simulink model "mainModel"  (R2024b)
settings: Solver=ode4  StartTime=0.0  StopTime=35000  FixedStep=0.1  RelTol=1e-3
values from neighbouring files (symbols this model uses):
  actuators = actuatorsConfig()    [main.m]
  constant = constantsConfig()    [main.m]
  control = controlConfig(data)    [main.m]
  MEKF = estimationConfig(sensors,simOpt)    [main.m]
  pert = pertConfig()    [main.m]
  sensors = sensorsConfig()    [main.m]
undefined symbols (not defined in the file or in its folder): Ab0, data, DiscIntNeverNeededParam, init
libraries: matrix_library x38, simulink x10, aerolibutil x7, simulink_extras x6, sharedtransform x1, dspinverses x1, dspfdesign x1, dspstat3 x1
(part 2 of 3)

== system mainModel/TRIAD/errorsTRIAD ==
  A_BN : Inport
  A_BN_est : Inport  Port=2
  w : Inport  Port=3
  w_estTRIAD : Inport  Port=4
  Minus1 : Sum  Inputs=+-
  Reshape : Reshape
  Scope : Scope
  Scope1 : Scope
  Scope2 : Scope
  Scope3 : Scope  NumInputPorts=2
  TRUE^t * SYM : Product  Multiplication=Matrix(*)
  To Workspace : ToWorkspace  VariableName=errTRIAD  SampleTime=-1
  Transpose : Math  Operator=transpose
  Zero-Order Hold : ZeroOrderHold  SampleTime=0.1
  Zero-Order Hold1 : ZeroOrderHold  SampleTime=0.1
  angle error : Subsystem
  wires:
  A_BN/1 -> Zero-Order Hold/1
  w/1 -> Zero-Order Hold1/1
  w_estTRIAD/1 -> Scope3/2, Minus1/2
  Minus1/1 -> Scope1/1
  TRUE^t * SYM/1 -> angle error/1(Aerr)
  angle error/1(theta_err) -> Reshape/1
  Transpose/1 -> TRUE^t * SYM/1
  A_BN_est/1 -> TRUE^t * SYM/2, Scope2/1
  Zero-Order Hold/1 -> Scope/1, Transpose/1
  Zero-Order Hold1/1 -> Scope3/1, Minus1/1
  Reshape/1 -> To Workspace/1

== system mainModel/angular rates estimation QUEST /angVelEstimation ==
  q_est : Inport
  Discrete-Time Integrator : DiscreteIntegrator  SampleTime=-1  ICPrevOutput=DiscIntNeverNeededParam  ICPrevScaledInput=DiscIntNeverNeededParam
  Gain : Gain  Gain=2
  Qmatrix : Subsystem  ReferencedSubsystem=Qmatrix
  Scope : Scope
  "[Q*] * q_dot" : Product  Multiplication=Matrix(*)
  pseudoInverseMatrix : Subsystem  ReferencedSubsystem=pseudoInverseMatrix
  w_est : Outport
  wires:
  q_est/1 -> Discrete-Time Integrator/1, Qmatrix/1
  Gain/1 -> Scope/1, w_est/1
  Discrete-Time Integrator/1 -> "[Q*] * q_dot"/2  "q_dot"
  "[Q*] * q_dot"/1 -> Gain/1
  Qmatrix/1 -> pseudoInverseMatrix/1
  pseudoInverseMatrix/1 -> "[Q*] * q_dot"/1

== system mainModel/angular rates estimation QUEST /svd ==
  K : Inport
  Dot Product : DotProduct  OutDataTypeStr=Inherit: Inherit via internal rule
  Gain : Gain  Gain=-1
  K * q : Product  Multiplication=Matrix(*)
  Memory : Memory  InitialCondition=init.q0
  Scope{,1..3} (4 alike) : Scope
  Subsystem Reference : Subsystem  ReferencedSubsystem=vecNorm
  Switch : Switch  Criteria=u2 > Threshold  SaturateOnIntegerOverflow=off  InputSameDT=off
  Terminator : Terminator
  To Workspace : ToWorkspace  VariableName=q_est_SVD  SampleTime=-1
  q_est : Outport
  wires:
  K/1 -> Scope1/1, K * q/1  "Kmatrix (4x4)"
  Subsystem Reference/2 -> Switch/1, Gain/1, Memory/1, Dot Product/1, Scope/1, Scope3/1, To Workspace/1, q_est/1  "q_optimal"
  Subsystem Reference/1 -> Terminator/1
  Memory/1 -> K * q/2, Dot Product/2  "qVec (4x1)"
  K * q/1 -> Subsystem Reference/1
  Dot Product/1 -> Switch/2
  Gain/1 -> Switch/3
  Switch/1 -> Scope2/1

== system mainModel/atmDrag/DRAG torque  ==
  rho : Inport
  velRel_B : Inport  Port=2
  w_B : Inport  Port=3
  Constant : Constant  Value=pert.drag.Nbvect
  Constant1 : Constant  Value=pert.drag.rF
  Constant2 : Constant  Value=pert.drag.A
  Relative velocity body : Subsystem
  To Workspace1 : ToWorkspace  VariableName=dragPertMatrix  SampleTime=-1
  dragForce : Subsystem
  dragTorque : Subsystem
  vecCrossOld : Subsystem  Commented=on
  DRAG : Outport
  wires:
  velRel_B/1 -> Relative velocity body/1(velRel_B)
  w_B/1 -> Relative velocity body/2(om_B)
  Constant1/1 -> Relative velocity body/3(rF), dragTorque/2(rFvect)
  Relative velocity body/1(vRelBody) -> dragForce/2(vRelBody)
  rho/1 -> dragForce/1(rho)
  Constant/1 -> dragForce/3(Nb)
  Constant2/1 -> dragForce/4(A)
  dragForce/1(F) -> dragTorque/1(Fvect)
  dragTorque/1(DRAG) -> DRAG/1
  dragTorque/2(dragMATRIX) -> To Workspace1/1

== system mainModel/atmDrag/density ==
  r_N : Inport
  Constant : Constant  Value=constant.Re
  Constant1 : Constant  Value=pert.drag.h0_vect
  Constant2 : Constant  Value=pert.drag.H_vect
  Constant4 : Constant  Value=pert.drag.rho0_vect
  Constant5 : Constant  Value=pert.drag.h0_vect
  Divide : Product  Inputs=*/
  Exp : Math
  Gain : Gain  Gain=-1
  Interpolation Using Prelookup : Interpolation_n-D  NumberOfTableDimensions=1  TableSource=Input port  InternalRulePriority=Speed
      settings: InputPortMap=u0,u1,p2
  Interpolation Using Prelookup1 : Interpolation_n-D  NumberOfTableDimensions=1  TableSource=Input port  InternalRulePriority=Speed
      settings: InputPortMap=u0,u1,p2
  Interpolation Using Prelookup2 : Interpolation_n-D  NumberOfTableDimensions=1  TableSource=Input port  InternalRulePriority=Speed
      settings: InputPortMap=u0,u1,p2
  Minus : Sum  Inputs=+-
  Minus1 : Sum  Inputs=+-
  Prelookup : PreLookup  BreakpointsDataSource=Input port  BreakpointsData=[10:10:110]  ExtrapMethod=Linear
      settings: InputPortMap=u0,p1
  Product : Product
  Subsystem Reference : Subsystem  ReferencedSubsystem=vecNorm
  Terminator : Terminator
  rho : Outport
  wires:
  r_N/1 -> Subsystem Reference/1
  Subsystem Reference/2 -> Terminator/1
  Subsystem Reference/1 -> Minus/1
  Constant/1 -> Minus/2
  Minus/1 -> Minus1/1, Prelookup/1  "h"
  Constant1/1 -> Prelookup/2
  Prelookup/1 -> Interpolation Using Prelookup/1, Interpolation Using Prelookup2/1, Interpolation Using Prelookup1/1
  Prelookup/2 -> Interpolation Using Prelookup/2, Interpolation Using Prelookup1/2, Interpolation Using Prelookup2/2
  Constant5/1 -> Interpolation Using Prelookup/3
  Constant2/1 -> Interpolation Using Prelookup1/3
  Constant4/1 -> Interpolation Using Prelookup2/3
  Interpolation Using Prelookup/1 -> Minus1/2
  Interpolation Using Prelookup1/1 -> Divide/2
  Minus1/1 -> Divide/1
  Divide/1 -> Gain/1
  Exp/1 -> Product/1
  Interpolation Using Prelookup2/1 -> Product/2
  Product/1 -> rho/1
  Gain/1 -> Exp/1

== system mainModel/atmDrag/relVel ==
  A_BN : Inport
  r_N : Inport  Port=2
  vel_N : Inport  Port=3
  A_BN * velRel_N : Product  Multiplication=Matrix(*)
  Add : Sum  Inputs=-+
  Constant : Constant  Value=[0;0;constant.we]  VectorParams1D=off
  Cross Product : matrix_library/Cross Product
  velRel_B : Outport
  wires:
  Constant/1 -> Cross Product/1
  r_N/1 -> Cross Product/2
  Cross Product/1 -> Add/1
  vel_N/1 -> Add/2
  Add/1 -> A_BN * velRel_N/2  "velRel_N"
  A_BN/1 -> A_BN * velRel_N/1
  A_BN * velRel_N/1 -> velRel_B/1

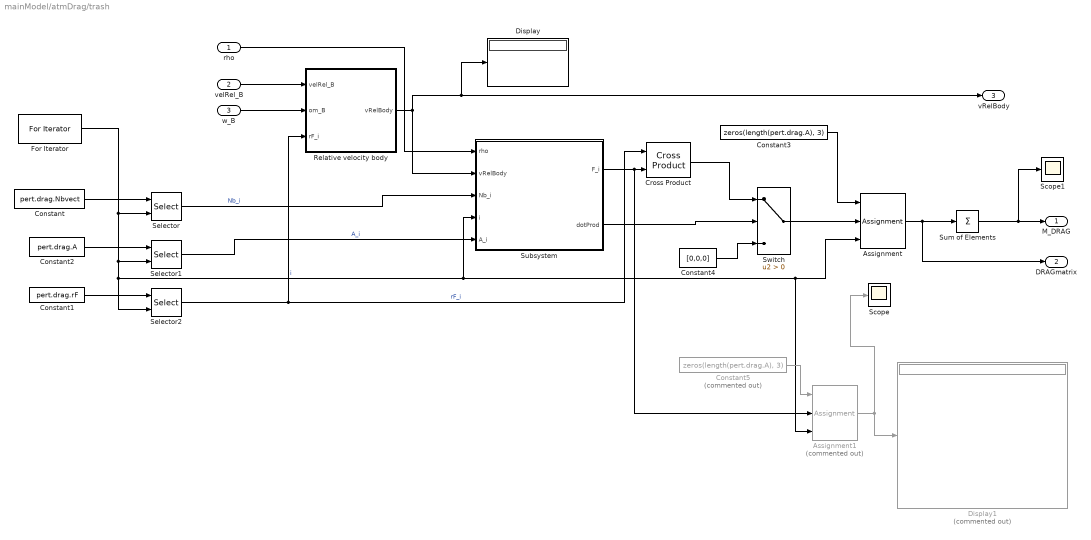
== system mainModel/atmDrag/trash ==
  rho : Inport
  velRel_B : Inport  Port=2
  w_B : Inport  Port=3
  Assignment : Assignment  NumberOfDimensions=2  DiagnosticForDimensions=Warning  IndexOptions=Index vector (port),Assign all  Indices=1,1  OutputSizes=1,1
  Assignment1 : Assignment  Commented=on  NumberOfDimensions=2  DiagnosticForDimensions=Warning  IndexOptions=Index vector (port),Assign all  Indices=1,1  OutputSizes=1,1
  Constant : Constant  Value=pert.drag.Nbvect
  Constant1 : Constant  Value=pert.drag.rF
  Constant2 : Constant  Value=pert.drag.A
  Constant3 : Constant  Value=zeros(length(pert.drag.A), 3)  VectorParams1D=off
  Constant4 : Constant  Value=[0,0,0]  VectorParams1D=off
  Constant5 : Constant  Commented=on  Value=zeros(length(pert.drag.A), 3)  VectorParams1D=off
  Cross Product : matrix_library/Cross Product
  Display : Display
  Display1 : Display  Commented=on
  For Iterator : ForIterator  IterationLimit=length(pert.drag.A)
  Relative velocity body : Subsystem
  Scope : Scope
  Scope1 : Scope
  Selector : Selector  NumberOfDimensions=2  InputPortWidth=3  IndexOptions=Index vector (port),Select all  Indices=[1 3],1  OutputSizes=1,1
  Selector1 : Selector  InputPortWidth=10  IndexOptions=Index vector (port)  Indices=[1 3]  OutputSizes=1
  Selector2 : Selector  NumberOfDimensions=2  InputPortWidth=3  IndexOptions=Index vector (port),Select all  Indices=[1 3],1  OutputSizes=1,1
  Subsystem : Subsystem
  Sum of Elements : Sum  Inputs=+  CollapseMode=Specified dimension
  Switch : Switch  Criteria=u2 > Threshold  SaturateOnIntegerOverflow=off  InputSameDT=off
  M_DRAG : Outport
  DRAGmatrix : Outport  Port=2
  vRelBody : Outport  Port=3
  wires:
  Constant/1 -> Selector/1
  Constant2/1 -> Selector1/1
  Constant1/1 -> Selector2/1
  Selector2/1 -> Relative velocity body/3(rF_i), Cross Product/1  "rF_i"
  For Iterator/1 -> Selector2/2, Subsystem/4(i), Assignment1/3, Assignment/3, Selector1/2, Selector/2  "i"
  Cross Product/1 -> Switch/1
  rho/1 -> Subsystem/1(rho)
  velRel_B/1 -> Relative velocity body/1(velRel_B)
  Selector/1 -> Subsystem/3(Nb_i)  "Nb_i"
  Selector1/1 -> Subsystem/5(A_i)  "A_i"
  Subsystem/1(F_i) -> Assignment1/2, Cross Product/2
  Assignment/1 -> Sum of Elements/1, DRAGmatrix/1
  Relative velocity body/1(vRelBody) -> Display/1, vRelBody/1, Subsystem/2(vRelBody)
  Sum of Elements/1 -> Scope1/1, M_DRAG/1
  Constant3/1 -> Assignment/1
  Subsystem/2(dotProd) -> Switch/2
  Constant4/1 -> Switch/3
  Switch/1 -> Assignment/2
  w_B/1 -> Relative velocity body/2(om_B)
  Constant5/1 -> Assignment1/1
  Assignment1/1 -> Scope/1, Display1/1

== system mainModel/attitudeDetermination_QUATERNION/QUEST ==
  S : Inport
  z : Inport  Port=2
  sigma : Inport  Port=3
  -z * [S-(sigma+1)*I]^-1 : Product  Multiplication=Matrix(*)
  Add : Sum
  Add1 : Sum
  Constant : Constant  Value=init.lambda0
  Constant1 : Constant  Value=eye(3)
  Gain : Gain  Gain=-1
  Gain1 : Gain  Gain=-1
  Product : Product
  Scope3 : Scope
  Subsystem Reference : Subsystem  ReferencedSubsystem=invertMatrix
  Subsystem Reference1 : Subsystem  ReferencedSubsystem=quat2DCM
  To Workspace : ToWorkspace  VariableName=q_est_QUESTgibbs  SampleTime=-1
  fix quat : Subsystem  ReferencedSubsystem=quatFix
  gibbs2quat : Subsystem  ReferencedSubsystem=gibbs2quat
  q_est : Outport
  wires:
  sigma/1 -> Add/1
  Add/1 -> Product/1  "sigma + 1"
  Constant1/1 -> Product/2
  Product/1 -> Gain/1
  Gain/1 -> Add1/2  "-(sigma+1)*I"
  S/1 -> Add1/1  "S"
  Subsystem Reference/1 -> -z * [S-(sigma+1)*I]^-1/1
  z/1 -> Gain1/1
  -z * [S-(sigma+1)*I]^-1/1 -> gibbs2quat/1  "gibbs_est"
  Gain1/1 -> -z * [S-(sigma+1)*I]^-1/2
  gibbs2quat/1 -> fix quat/1  "q_prev"
  fix quat/1 -> Subsystem Reference1/1, To Workspace/1, q_est/1
  Constant/1 -> Add/2
  Add1/1 -> Subsystem Reference/1
  Subsystem Reference1/1 -> Scope3/1

== system mainModel/attitudeDetermination_QUATERNION/QUEST V2 ==
  z : Inport
  sigma : Inport  Port=2
  S : Inport  Port=3
  Add : Sum
  Constant : Constant  Value=eye(3)
  Constant1 : Constant  Value=init.lambda0
  Minus : Sum  Inputs=+-
  Product : Product
  Product1 : Product  Multiplication=Matrix(*)
  Scope1 : Scope
  Subsystem Reference : Subsystem  ReferencedSubsystem=matrixDeterminant
  Subsystem Reference2 : Subsystem  ReferencedSubsystem=vecNorm
  Subsystem Reference3 : Subsystem  ReferencedSubsystem=quat2DCM
  Terminator : Terminator
  To Workspace1 : ToWorkspace  VariableName=q_est_QUESTadj  SampleTime=-1
  Vector Concatenate : Concatenate
  adjointMatrix : Subsystem
  q_est : Outport
  wires:
  sigma/1 -> Add/1
  Add/1 -> Product/2  "rho"
  Constant/1 -> Product/1
  Constant1/1 -> Add/2
  Product/1 -> Minus/1  "rho*I"
  S/1 -> Minus/2
  Minus/1 -> Subsystem Reference/1, adjointMatrix/1(A)
  z/1 -> Product1/2
  Product1/1 -> Vector Concatenate/1
  Subsystem Reference/1 -> Vector Concatenate/2
  Vector Concatenate/1 -> Subsystem Reference2/1
  Subsystem Reference2/2 -> To Workspace1/1, q_est/1, Subsystem Reference3/1
  Subsystem Reference3/1 -> Scope1/1
  adjointMatrix/1(Out1) -> Product1/1
  Subsystem Reference2/1 -> Terminator/1

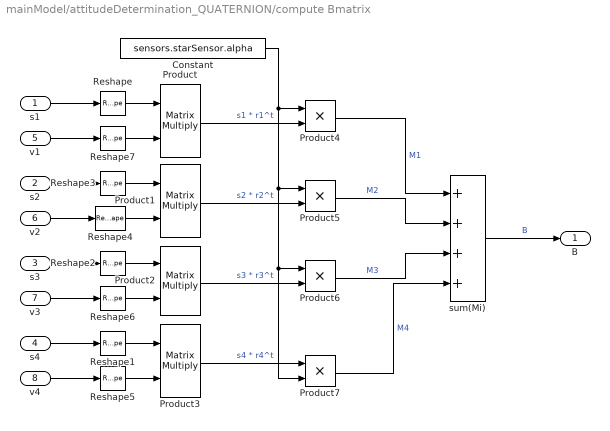
== system mainModel/attitudeDetermination_QUATERNION/compute Bmatrix ==
  s1 : Inport
  s2 : Inport  Port=2
  s3 : Inport  Port=3
  s4 : Inport  Port=4
  v1 : Inport  Port=5
  v2 : Inport  Port=6
  v3 : Inport  Port=7
  v4 : Inport  Port=8
  Constant : Constant  Value=sensors.starSensor.alpha
  Product{,1..3} (4 alike) : Product  Multiplication=Matrix(*)
  Product{4..7} (4 alike) : Product
  Reshape{,1..3} (4 alike) : Reshape  OutputDimensionality=Column vector (2-D)
  Reshape{4..7} (4 alike) : Reshape  OutputDimensionality=Row vector (2-D)
  sum(Mi) : Sum  Inputs=++++
  B : Outport
  wires:
  sum(Mi)/1 -> B/1  "B"
  Product/1 -> Product4/2  "s1 * r1^t"
  Constant/1 -> Product4/1, Product5/1, Product7/2, Product6/1
  Product1/1 -> Product5/2  "s2 * r2^t"
  Product2/1 -> Product6/2  "s3 * r3^t"
  Product3/1 -> Product7/1  "s4 * r4^t"
  Product4/1 -> sum(Mi)/1  "M1"
  Product6/1 -> sum(Mi)/3  "M3"
  Product5/1 -> sum(Mi)/2  "M2"
  Reshape4/1 -> Product1/2
  Reshape1/1 -> Product3/1
  Reshape/1 -> Product/1
  Reshape2/1 -> Product2/1
  Reshape6/1 -> Product2/2
  Reshape7/1 -> Product/2
  Reshape5/1 -> Product3/2
  v4/1 -> Reshape5/1
  v2/1 -> Reshape4/1
  v1/1 -> Reshape7/1
  s1/1 -> Reshape/1
  Reshape3/1 -> Product1/1
  v3/1 -> Reshape6/1
  s4/1 -> Reshape1/1
  s3/1 -> Reshape2/1
  Product7/1 -> sum(Mi)/4  "M4"
  s2/1 -> Reshape3/1

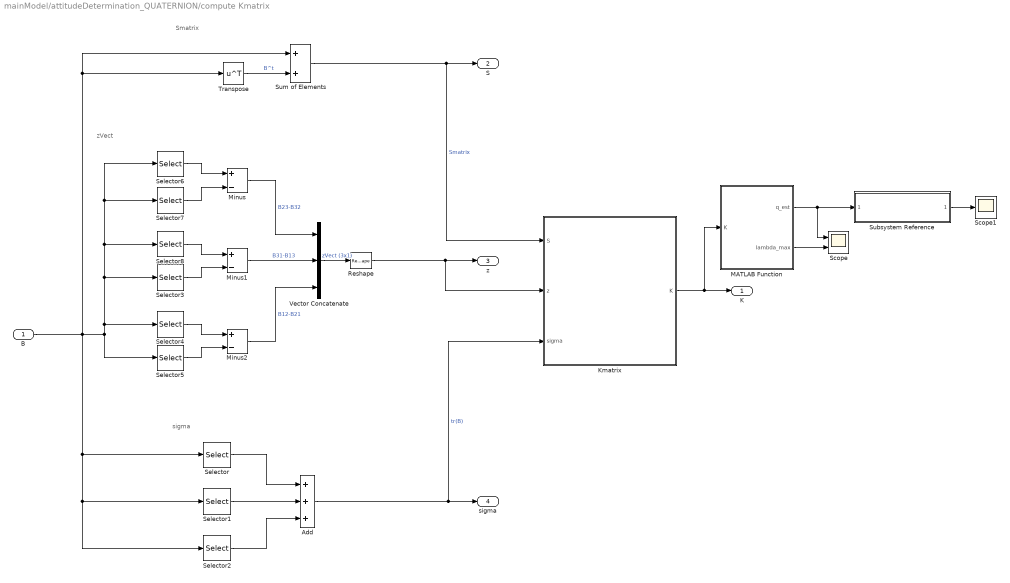
== system mainModel/attitudeDetermination_QUATERNION/compute Kmatrix ==
  note: Smatrix
  note: zVect
  note: sigma
  B : Inport
  Add : Sum  Inputs=+++
  Kmatrix : Subsystem
  MATLAB Function : MATLAB Function  TreatAsAtomicUnit=on
  Minus : Sum  Inputs=+-
  Minus1 : Sum  Inputs=+-
  Minus2 : Sum  Inputs=+-
  Reshape : Reshape  OutputDimensionality=Column vector (2-D)
  Scope : Scope  NumInputPorts=2
  Scope1 : Scope
  Selector : Selector  NumberOfDimensions=2  InputPortWidth=3  IndexOptions=Index vector (dialog),Index vector (dialog)  Indices=1,1  OutputSizes=1,1
  Selector1 : Selector  NumberOfDimensions=2  InputPortWidth=3  IndexOptions=Index vector (dialog),Index vector (dialog)  Indices=2,2  OutputSizes=1,1
  Selector2 : Selector  NumberOfDimensions=2  InputPortWidth=3  IndexOptions=Index vector (dialog),Index vector (dialog)  Indices=3,3  OutputSizes=1,1
  Selector3 : Selector  NumberOfDimensions=2  InputPortWidth=3  IndexOptions=Index vector (dialog),Index vector (dialog)  Indices=1,3  OutputSizes=1,1
  Selector4 : Selector  NumberOfDimensions=2  InputPortWidth=3  IndexOptions=Index vector (dialog),Index vector (dialog)  Indices=1,2  OutputSizes=1,1
  Selector5 : Selector  NumberOfDimensions=2  InputPortWidth=3  IndexOptions=Index vector (dialog),Index vector (dialog)  Indices=2,1  OutputSizes=1,1
  Selector6 : Selector  NumberOfDimensions=2  InputPortWidth=3  IndexOptions=Index vector (dialog),Index vector (dialog)  Indices=2,3  OutputSizes=1,1
  Selector7 : Selector  NumberOfDimensions=2  InputPortWidth=3  IndexOptions=Index vector (dialog),Index vector (dialog)  Indices=3,2  OutputSizes=1,1
  Selector8 : Selector  NumberOfDimensions=2  InputPortWidth=3  IndexOptions=Index vector (dialog),Index vector (dialog)  Indices=3,1  OutputSizes=1,1
  Subsystem Reference : Subsystem  ReferencedSubsystem=quat2DCM
  Sum of Elements : Sum
  Transpose : Math  Operator=transpose
  Vector Concatenate : Concatenate  NumInputs=3
  K : Outport
  S : Outport  Port=2
  z : Outport  Port=3
  sigma : Outport  Port=4
  wires:
  Reshape/1 -> Kmatrix/2(z), z/1
  Kmatrix/1(K) -> MATLAB Function/1(K), K/1
  Add/1 -> Kmatrix/3(sigma), sigma/1  "tr(B)"
  Selector2/1 -> Add/3
  Selector/1 -> Add/1
  Selector1/1 -> Add/2
  Vector Concatenate/1 -> Reshape/1  "zVect (3x1)"
  Minus2/1 -> Vector Concatenate/3  "B12-B21"
  Minus/1 -> Vector Concatenate/1  "B23-B32"
  Minus1/1 -> Vector Concatenate/2  "B31-B13"
  Selector4/1 -> Minus2/1
  Selector5/1 -> Minus2/2
  Selector8/1 -> Minus1/1
  Selector3/1 -> Minus1/2
  Selector7/1 -> Minus/2
  Selector6/1 -> Minus/1
  Transpose/1 -> Sum of Elements/2  "B^t"
  B/1 -> Selector2/1, Selector1/1, Selector/1, Selector3/1, Selector8/1, Selector7/1, Selector6/1, Selector4/1, Selector5/1, Transpose/1, Sum of Elements/1
  Sum of Elements/1 -> S/1, Kmatrix/1(S)  "Smatrix"
  MATLAB Function/1(q_est) -> Subsystem Reference/1, Scope/1
  MATLAB Function/2(lambda_max) -> Scope/2
  Subsystem Reference/1 -> Scope1/1

== system mainModel/attitudeDetermination_QUATERNION/matlaFunction for Davenport's q-method ==
  K : Inport
  MATLAB Function : MATLAB Function  TreatAsAtomicUnit=on
  Reshape : Reshape
  Reshape1 : Reshape
  To Workspace : ToWorkspace  VariableName=lambdaMax_DavqMethod  SampleTime=-1
  To Workspace3 : ToWorkspace  VariableName=q_est_DavqMethod  SampleTime=-1
  q_est : Outport
  lambda_max : Outport  Port=2
  wires:
  MATLAB Function/1(q_est) -> q_est/1, Reshape1/1
  K/1 -> MATLAB Function/1(K)
  MATLAB Function/2(lambda_max) -> lambda_max/1, Reshape/1
  Reshape/1 -> To Workspace/1
  Reshape1/1 -> To Workspace3/1

== system mainModel/attitudeDetermination_QUATERNION/quest - shuster ==
  note: compute MAX eigenvalue
  S : Inport
  z : Inport  Port=2
  Constant : Constant  Value=init.lambda0
  Reshape : Reshape
  Scope1 : Scope
  Scope2 : Scope
  Subsystem Reference : Subsystem  ReferencedSubsystem=quat2DCM
  To Workspace : ToWorkspace  VariableName=lambdaMax_QUESTshuster  SampleTime=-1
  To Workspace2 : ToWorkspace  VariableName=q_est_QUESTshuster  SampleTime=-1
  compute optimal quaternion : Subsystem
  mewton method step-two : Subsystem  Commented=on
  newton method step-one : Subsystem
  shuster parameters : Subsystem
  q_est : Outport
  lambda : Outport  Port=2
  wires:
  compute optimal quaternion/1(q_est) -> Scope1/1, To Workspace2/1, Subsystem Reference/1, q_est/1
  Reshape/1 -> compute optimal quaternion/1(lambda), lambda/1, To Workspace/1
  S/1 -> compute optimal quaternion/5(S), shuster parameters/1(S)  "S"
  z/1 -> compute optimal quaternion/6(z), shuster parameters/2(z)  "z"
  shuster parameters/6(k) -> compute optimal quaternion/3(k)
  shuster parameters/7(Delta) -> compute optimal quaternion/4(Delta)
  Subsystem Reference/1 -> Scope2/1
  newton method step-one/1(lambda1) -> Reshape/1
  Constant/1 -> newton method step-one/1(lambda)
  shuster parameters/4(d) -> newton method step-one/6(d)
  shuster parameters/3(c) -> newton method step-one/5(c)
  shuster parameters/2(b) -> newton method step-one/4(b)
  shuster parameters/1(a) -> newton method step-one/3(a)
  shuster parameters/5(sigma) -> newton method step-one/2(sigma), compute optimal quaternion/2(sigma)

== system mainModel/attitudeError/angle error ==
  Aerr : Inport
  Acos : Trigonometry  Operator=acos
  Add : Sum  Inputs=+++
  Constant : Constant
  Gain : Gain  Gain=1/2
  Minus1 : Sum  Inputs=+-
  Radians to Degrees : simulink_extras/Transformations/Radians to Degrees
  Selector : Selector  NumberOfDimensions=2  InputPortWidth=3  IndexOptions=Index vector (dialog),Index vector (dialog)  Indices=1,1  OutputSizes=1,1
  Selector1 : Selector  NumberOfDimensions=2  InputPortWidth=3  IndexOptions=Index vector (dialog),Index vector (dialog)  Indices=2,2  OutputSizes=1,1
  Selector2 : Selector  NumberOfDimensions=2  InputPortWidth=3  IndexOptions=Index vector (dialog),Index vector (dialog)  Indices=3,3  OutputSizes=1,1
  theta_err : Outport
  wires:
  Aerr/1 -> Selector2/1, Selector/1, Selector1/1
  Gain/1 -> Acos/1
  Selector1/1 -> Add/2
  Add/1 -> Minus1/1  "tr(Aerr)"
  Constant/1 -> Minus1/2
  Selector2/1 -> Add/3
  Minus1/1 -> Gain/1
  Selector/1 -> Add/1
  Acos/1 -> Radians to Degrees/1
  Radians to Degrees/1 -> theta_err/1

== system mainModel/attitudeError1/angle error ==
  Aerr : Inport
  Acos : Trigonometry  Operator=acos
  Add : Sum  Inputs=+++
  Constant : Constant
  Gain : Gain  Gain=1/2
  Minus1 : Sum  Inputs=+-
  Radians to Degrees : simulink_extras/Transformations/Radians to Degrees
  Reshape : Reshape
  Selector : Selector  NumberOfDimensions=2  InputPortWidth=3  IndexOptions=Index vector (dialog),Index vector (dialog)  Indices=1,1  OutputSizes=1,1
  Selector1 : Selector  NumberOfDimensions=2  InputPortWidth=3  IndexOptions=Index vector (dialog),Index vector (dialog)  Indices=2,2  OutputSizes=1,1
  Selector2 : Selector  NumberOfDimensions=2  InputPortWidth=3  IndexOptions=Index vector (dialog),Index vector (dialog)  Indices=3,3  OutputSizes=1,1
  theta_err : Outport
  wires:
  Aerr/1 -> Selector2/1, Selector/1, Selector1/1
  Gain/1 -> Acos/1
  Selector1/1 -> Add/2
  Add/1 -> Minus1/1  "tr(Aerr)"
  Constant/1 -> Minus1/2
  Selector2/1 -> Add/3
  Minus1/1 -> Gain/1
  Selector/1 -> Add/1
  Acos/1 -> Radians to Degrees/1
  Radians to Degrees/1 -> Reshape/1
  Reshape/1 -> theta_err/1

== system mainModel/basicMagModel/mHat ==
  we : Inport
  magAxAngle : Inport  Port=2
  Clock : Clock
  Cos : Trigonometry
  Cos1 : Trigonometry  Operator=cos
  Cos2 : Trigonometry
  Cos3 : Trigonometry  Operator=cos
  Product : Product
  Product1 : Product
  Product2 : Product
  Vector Concatenate : Concatenate  NumInputs=3
  mHat : Outport
  wires:
  Vector Concatenate/1 -> mHat/1
  Clock/1 -> Product/2
  Product/1 -> Cos2/1, Cos1/1
  we/1 -> Product/1
  magAxAngle/1 -> Cos/1, Cos3/1
  Product1/1 -> Vector Concatenate/2
  Product2/1 -> Vector Concatenate/1
  Cos3/1 -> Vector Concatenate/3
  Cos/1 -> Product1/2, Product2/2
  Cos1/1 -> Product2/1
  Cos2/1 -> Product1/1

== system mainModel/errorsMEKF/angle error ==
  Aerr : Inport
  Acos : Trigonometry  Operator=acos
  Add : Sum  Inputs=+++
  Constant : Constant
  Gain : Gain  Gain=1/2
  Minus1 : Sum  Inputs=+-
  Radians to Degrees : simulink_extras/Transformations/Radians to Degrees
  Reshape : Reshape
  Selector : Selector  NumberOfDimensions=2  InputPortWidth=3  IndexOptions=Index vector (dialog),Index vector (dialog)  Indices=1,1  OutputSizes=1,1
  Selector1 : Selector  NumberOfDimensions=2  InputPortWidth=3  IndexOptions=Index vector (dialog),Index vector (dialog)  Indices=2,2  OutputSizes=1,1
  Selector2 : Selector  NumberOfDimensions=2  InputPortWidth=3  IndexOptions=Index vector (dialog),Index vector (dialog)  Indices=3,3  OutputSizes=1,1
  theta_err : Outport
  wires:
  Aerr/1 -> Selector2/1, Selector/1, Selector1/1
  Gain/1 -> Acos/1
  Selector1/1 -> Add/2
  Add/1 -> Minus1/1  "tr(Aerr)"
  Constant/1 -> Minus1/2
  Selector2/1 -> Add/3
  Minus1/1 -> Gain/1
  Selector/1 -> Add/1
  Acos/1 -> Radians to Degrees/1
  Radians to Degrees/1 -> Reshape/1
  Reshape/1 -> theta_err/1

== system mainModel/errorsQUEST/angle error ==
  Aerr : Inport
  Acos : Trigonometry  Operator=acos
  Add : Sum  Inputs=+++
  Constant : Constant
  Gain : Gain  Gain=1/2
  Minus1 : Sum  Inputs=+-
  Radians to Degrees : simulink_extras/Transformations/Radians to Degrees
  Reshape : Reshape
  Selector : Selector  NumberOfDimensions=2  InputPortWidth=3  IndexOptions=Index vector (dialog),Index vector (dialog)  Indices=1,1  OutputSizes=1,1
  Selector1 : Selector  NumberOfDimensions=2  InputPortWidth=3  IndexOptions=Index vector (dialog),Index vector (dialog)  Indices=2,2  OutputSizes=1,1
  Selector2 : Selector  NumberOfDimensions=2  InputPortWidth=3  IndexOptions=Index vector (dialog),Index vector (dialog)  Indices=3,3  OutputSizes=1,1
  theta_err : Outport
  wires:
  Aerr/1 -> Selector2/1, Selector/1, Selector1/1
  Gain/1 -> Acos/1
  Selector1/1 -> Add/2
  Add/1 -> Minus1/1  "tr(Aerr)"
  Constant/1 -> Minus1/2
  Selector2/1 -> Add/3
  Minus1/1 -> Gain/1
  Selector/1 -> Add/1
  Acos/1 -> Radians to Degrees/1
  Radians to Degrees/1 -> Reshape/1
  Reshape/1 -> theta_err/1

== system mainModel/magnetometerModel/Subsystem2 ==
  Clock2 : Clock
  Zero-Order Hold : ZeroOrderHold  SampleTime=sensors.magnetometer.sampleTime
  clock : Outport
  wires:
  Zero-Order Hold/1 -> clock/1
  Clock2/1 -> Zero-Order Hold/1

== system mainModel/orthoNormalization/orthonormalization ==
  A : Inport
  Add : Sum  Inputs=+-
  Gain : Gain  Gain=3/2
  Gain1 : Gain  Gain=1/2
  Product1 : Product  Inputs=3  Multiplication=Matrix(*)
  Transpose : Math  Operator=transpose
  Anew : Outport
  wires:
  Gain/1 -> Add/1
  Transpose/1 -> Product1/2  "A^t"
  Product1/1 -> Gain1/1
  Gain1/1 -> Add/2
  Add/1 -> Anew/1  "Anew"
  A/1 -> Product1/3, Transpose/1, Product1/1, Gain/1

== system mainModel/positionVect/direction ==
  theta : Inport
  i : Inport  Port=2
  Cos : Trigonometry  Operator=cos
  Cos1 : Trigonometry  Operator=cos
  Product : Product
  Product1 : Product
  Sin : Trigonometry
  Sin1 : Trigonometry
  Vector Concatenate : Concatenate  NumInputs=3
  dir : Outport
  wires:
  Product/1 -> Vector Concatenate/3
  i/1 -> Sin1/1, Cos1/1
  Cos1/1 -> Product1/2
  theta/1 -> Sin/1, Cos/1
  Cos/1 -> Vector Concatenate/1
  Product1/1 -> Vector Concatenate/2
  Sin/1 -> Product1/1, Product/1
  Sin1/1 -> Product/2
  Vector Concatenate/1 -> dir/1  "dir"

== system mainModel/positionVect/value ==
  theta : Inport
  Add : Sum
  Add1 : Sum  Inputs=+-
  Constant1 : Constant
  Constant2 : Constant  Value=data.e
  Constant3 : Constant
  Cos : Trigonometry  Operator=cos
  Divide : Product  Inputs=*/
  Gain : Gain  Gain=data.e
  Gain1 : Gain  Gain=data.a
  Square : Math  Operator=square
  r : Outport
  wires:
  Constant2/1 -> Square/1
  Cos/1 -> Gain/1
  Gain/1 -> Add/2
  Add1/1 -> Gain1/1
  Square/1 -> Add1/2
  Gain1/1 -> Divide/1
  Constant1/1 -> Add/1
  Add/1 -> Divide/2
  Constant3/1 -> Add1/1
  Divide/1 -> r/1  "r"
  theta/1 -> Cos/1

== system mainModel/reactionWheel/backup ==
  controlTq : Inport
  w_corr : Inport  Port=2
  Band-Limited White Noise : simulink/Sources/Band-Limited White Noise  Commented=on  Cov=[0.1]  Ts=0.1  seed=[23341]
  Constant : Constant  Value=0
  Constant1 : Constant  Value=0
  Discrete-Time Integrator : DiscreteIntegrator  SampleTime=-1  LimitOutput=on  UpperSaturationLimit=actuators.wheel.maxMomentum  LowerSaturationLimit=-actuators.wheel.maxMomentum  ICPrevOutput=DiscIntNeverNeededParam  ICPrevScaledInput=DiscIntNeverNeededParam
  Quantizer : Quantizer  Commented=through
  Rate Limiter : RateLimiter  RisingSlewLimit=0.01  FallingSlewLimit=-0.01  SampleTimeMode=inherited
  Rate Limiter1 : RateLimiter  RisingSlewLimit=0.01  FallingSlewLimit=-0.01  SampleTimeMode=inherited
  Saturation : Saturate
  Selector : Selector  InputPortWidth=3  IndexOptions=Index vector (dialog)  Indices=3  OutputSizes=1
  Sum : Sum  Inputs=+++
  Vector Concatenate : Concatenate  NumInputs=3
  hDotWheel : Outport
  hWheel : Outport  Port=2
  wires:
  Sum/1 -> Saturation/1
  Rate Limiter/1 -> hDotWheel/1
  Vector Concatenate/1 -> Sum/1  "hDotWheel"
  Constant/1 -> Vector Concatenate/1
  Saturation/1 -> Rate Limiter/1, Discrete-Time Integrator/1
  Band-Limited White Noise/1 -> Sum/2
  Quantizer/1 -> Selector/1
  controlTq/1 -> Quantizer/1
  Constant1/1 -> Vector Concatenate/2
  Discrete-Time Integrator/1 -> Rate Limiter1/1  "hWheel"
  Selector/1 -> Vector Concatenate/3
  Rate Limiter1/1 -> hWheel/1

== system mainModel/ref Attitude/Subsystem ==
  theta : Inport
  Constant1 : Constant  Value=[0,0,1]  VectorParams1D=off
  Constant2 : Constant  Value=0
  Cos : Trigonometry  Operator=cos
  Cos1 : Trigonometry
  Gain1 : Gain  Gain=-1
  Reshape : Reshape  OutputDimensionality=Row vector (2-D)
  Reshape1 : Reshape  OutputDimensionality=Row vector (2-D)
  Vector Concatenate : Concatenate  NumInputs=3
  Vector Concatenate1 : Concatenate  NumInputs=3
  Vector Concatenate2 : Concatenate  NumInputs=3  Mode=Multidimensional array
  R_theta : Outport
  wires:
  Reshape/1 -> Vector Concatenate2/1
  Vector Concatenate1/1 -> Reshape1/1
  Constant1/1 -> Vector Concatenate2/3
  Cos/1 -> Vector Concatenate1/2, Vector Concatenate/1
  theta/1 -> Cos1/1, Cos/1
  Constant2/1 -> Vector Concatenate/3, Vector Concatenate1/3
  Vector Concatenate/1 -> Reshape/1
  Cos1/1 -> Gain1/1, Vector Concatenate/2
  Reshape1/1 -> Vector Concatenate2/2
  Gain1/1 -> Vector Concatenate1/1
  Vector Concatenate2/1 -> R_theta/1

== system mainModel/ref Attitude/Subsystem1 ==
  Constant : Constant  Value=data.i
  Constant1 : Constant  Value=[1,0,0]  VectorParams1D=off
  Constant2 : Constant  Value=0
  Cos : Trigonometry  Operator=cos
  Cos1 : Trigonometry
  Gain1 : Gain  Gain=-1
  Reshape : Reshape  OutputDimensionality=Row vector (2-D)
  Reshape1 : Reshape  OutputDimensionality=Row vector (2-D)
  Vector Concatenate : Concatenate  NumInputs=3
  Vector Concatenate1 : Concatenate  NumInputs=3
  Vector Concatenate2 : Concatenate  NumInputs=3  Mode=Multidimensional array
  R_i : Outport
  wires:
  Vector Concatenate1/1 -> Reshape1/1
  Vector Concatenate/1 -> Reshape/1
  Reshape1/1 -> Vector Concatenate2/2
  Vector Concatenate2/1 -> R_i/1
  Constant/1 -> Cos1/1, Cos/1
  Constant1/1 -> Vector Concatenate2/1
  Reshape/1 -> Vector Concatenate2/3
  Gain1/1 -> Vector Concatenate/2
  Cos1/1 -> Vector Concatenate1/3, Gain1/1
  Cos/1 -> Vector Concatenate/3, Vector Concatenate1/2
  Constant2/1 -> Vector Concatenate1/1, Vector Concatenate/1

== system mainModel/starSensorModel/Subsystem ==
  Clock2 : Clock
  Zero-Order Hold : ZeroOrderHold  SampleTime=sensors.starSensor.sampleTime
  clock : Outport
  wires:
  Zero-Order Hold/1 -> clock/1
  Clock2/1 -> Zero-Order Hold/1

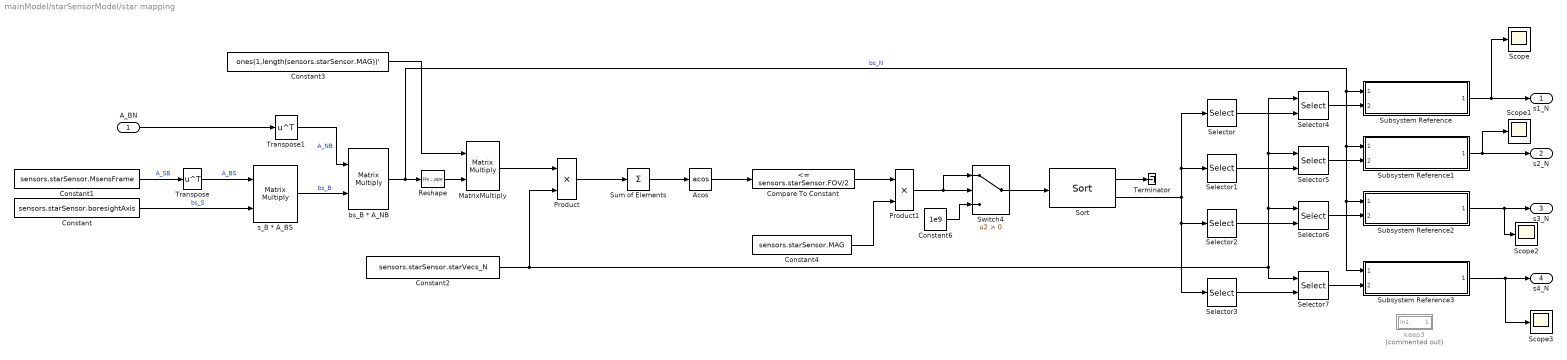
== system mainModel/starSensorModel/star mapping ==
  A_BN : Inport
  Acos : Trigonometry  Operator=acos
  Compare To Constant : simulink/Logic and Bit Operations/Compare To Constant  relop=<=  const=sensors.starSensor.FOV/2  OutDataTypeStr=boolean
  Constant : Constant  Value=sensors.starSensor.boresightAxis
  Constant1 : Constant  Value=sensors.starSensor.MsensFrame
  Constant2 : Constant  Value=sensors.starSensor.starVecs_N
  Constant3 : Constant  Value=ones(1,length(sensors.starSensor.MAG))'  VectorParams1D=off
  Constant4 : Constant  Value=sensors.starSensor.MAG
  Constant6 : Constant  Value=1e9
  MatrixMultiply : Product  Multiplication=Matrix(*)
  Product : Product
  Product1 : Product
  Reshape : Reshape  OutputDimensionality=Row vector (2-D)
  Scope{,1..3} (4 alike) : Scope
  Selector : Selector  InputPortWidth=length(sensors.starSensor.MAG)  IndexOptions=Index vector (dialog)  Indices=1  OutputSizes=1
  Selector1 : Selector  InputPortWidth=length(sensors.starSensor.MAG)  IndexOptions=Index vector (dialog)  Indices=2  OutputSizes=1
  Selector2 : Selector  InputPortWidth=length(sensors.starSensor.MAG)  IndexOptions=Index vector (dialog)  Indices=3  OutputSizes=1
  Selector3 : Selector  InputPortWidth=length(sensors.starSensor.MAG)  IndexOptions=Index vector (dialog)  Indices=4  OutputSizes=1
  Selector{4..7} (4 alike) : Selector  NumberOfDimensions=2  InputPortWidth=3  IndexOptions=Index vector (port),Select all  Indices=[1 3],1  OutputSizes=1,1
  Sort : dspstat3/Sort  otype=Value and Index  dir=Ascending  sortAlg=Quick sort  roundingMode=Floor  overflowMode=off  accumDataTypeStr=Inherit: Same as product output  accumLastDataTypeStr=Inherit: Same as product output
  Subsystem Reference{,1..3} (4 alike) : Subsystem  ReferencedSubsystem=keepWhileInFOV
  Sum of Elements : Sum  Inputs=+  CollapseMode=Specified dimension  CollapseDim=2
  Switch4 : Switch  Criteria=u2 > Threshold  SaturateOnIntegerOverflow=off  InputSameDT=off
  Terminator : Terminator
  Transpose : Math  Operator=transpose
  Transpose1 : Math  Operator=transpose
  bs_B * A_NB : Product  Multiplication=Matrix(*)
  keep3 : Subsystem  Commented=on
  s_B * A_BS : Product  Multiplication=Matrix(*)
  s1_N : Outport
  s2_N : Outport  Port=2
  s3_N : Outport  Port=3
  s4_N : Outport  Port=4
  wires:
  Constant/1 -> s_B * A_BS/2  "bs_S"
  Constant1/1 -> Transpose/1  "A_SB"
  Transpose/1 -> s_B * A_BS/1  "A_BS"
  s_B * A_BS/1 -> bs_B * A_NB/2  "bs_B"
  Product/1 -> Sum of Elements/1
  Acos/1 -> Compare To Constant/1
  Constant4/1 -> Product1/2
  A_BN/1 -> Transpose1/1
  Sum of Elements/1 -> Acos/1
  bs_B * A_NB/1 -> Subsystem Reference3/1, Subsystem Reference2/1, Subsystem Reference1/1, Subsystem Reference/1, Reshape/1  "bs_N"
  Sort/2 -> Selector3/1, Selector2/1, Selector/1, Selector1/1
  Selector3/1 -> Selector7/2
  Selector2/1 -> Selector6/2
  Selector1/1 -> Selector5/2
  Selector/1 -> Selector4/2
  Transpose1/1 -> bs_B * A_NB/1  "A_NB"
  Constant3/1 -> MatrixMultiply/1
  MatrixMultiply/1 -> Product/1
  Constant2/1 -> Product/2, Selector4/1, Selector5/1, Selector6/1, Selector7/1
  Reshape/1 -> MatrixMultiply/2
  Compare To Constant/1 -> Product1/1
  Product1/1 -> Switch4/1, Switch4/2
  Constant6/1 -> Switch4/3
  Switch4/1 -> Sort/1
  Sort/1 -> Terminator/1
  Selector4/1 -> Subsystem Reference/2
  Subsystem Reference/1 -> Scope/1, s1_N/1
  Selector7/1 -> Subsystem Reference3/2
  Selector6/1 -> Subsystem Reference2/2
  Selector5/1 -> Subsystem Reference1/2
  Subsystem Reference2/1 -> Scope2/1, s3_N/1
  Subsystem Reference3/1 -> Scope3/1, s4_N/1
  Subsystem Reference1/1 -> Scope1/1, s2_N/1

== system mainModel/thetaOrbit/theta_dot ==
  note: approximation
  theta : Inport
  Add : Sum
  Constant : Constant  Value=data.e
  Constant1 : Constant
  Constant2 : Constant  Value=3/2
  Constant3 : Constant  Value=data.n_sc
  Constant4 : Constant
  Cos : Trigonometry  Operator=cos
  Divide : Product  Inputs=*/
  Gain : Gain  Gain=data.e
  Power : Math  Operator=pow
  Power1 : Math  Operator=square
  Product : Product
  Square : Math  Operator=square
  Subtract : Sum  Inputs=+-
  theta_dot : Outport
  wires:
  Divide/1 -> theta_dot/1
  Power/1 -> Divide/2
  Constant/1 -> Square/1
  Constant1/1 -> Subtract/1
  Subtract/1 -> Power/1
  Constant2/1 -> Power/2
  theta/1 -> Cos/1
  Cos/1 -> Gain/1
  Gain/1 -> Add/2
  Add/1 -> Power1/1
  Power1/1 -> Product/2
  Constant3/1 -> Product/1
  Product/1 -> Divide/1
  Square/1 -> Subtract/2
  Constant4/1 -> Add/1

== system mainModel/MEKF ESTIMATION/CORRECTION/COVARIANCE MATRIX ==
  note: % aggiornamento matrice covarianza: formula Joseph
      | P_corr = (eye(6) - K * H) * P_pred * (eye(6) - K * H)' + K * R * K';
      | P_corr = 0.5 * (P_corr + P_corr'); % Simmetria
      | min_cov = 1e-10; % Valore minimo di incertezza
      | for i = 1:6
      | if P_corr(i,i) < min_cov
      | P_corr(i,i) = min_cov;
      | end
      | end
  K : Inport
  H : Inport  Port=2
  P_pred : Inport  Port=3
  Add1 : Sum
  Constant : Constant  Value=MEKF.R
  Constant1 : Constant  Value=eye(6)
  K * H : Product  Multiplication=Matrix(*)
  K * R * K' : Product  Inputs=3  Multiplication=Matrix(*)
  MatrixMultiply3 : Product  Inputs=3  Multiplication=Matrix(*)
  Transpose : Math  Operator=transpose
  Transpose1 : Math  Operator=transpose
  eye(6) - (K * H) : Sum  Inputs=+-
  P_corr : Outport
  wires:
  Constant/1 -> K * R * K'/2
  K/1 -> Transpose/1, K * R * K'/1, K * H/1
  Transpose/1 -> K * R * K'/3
  Constant1/1 -> eye(6) - (K * H)/1
  H/1 -> K * H/2
  K * H/1 -> eye(6) - (K * H)/2
  eye(6) - (K * H)/1 -> Transpose1/1, MatrixMultiply3/1
  P_pred/1 -> MatrixMultiply3/2
  Transpose1/1 -> MatrixMultiply3/3
  MatrixMultiply3/1 -> Add1/1
  K * R * K'/1 -> Add1/2
  Add1/1 -> P_corr/1

== system mainModel/MEKF ESTIMATION/MEASUREMENT/KALMAN GAIN ==
  note: %% kalman gain (K)
      | % S = H * P_pred * H' + R;
      | % epsilon = 1e-12;
      | % S_reg = S + eye(size(S)) * epsilon;
      | % K = (P_pred * H') / S_reg;
      | % 1. Calcoliamo S (Denominatore) e Num_K (Numeratore) separati
      | S = H * P_pred * H' + R;
      | Num_K = P_pred * H';
      |
      | S = S + eye(size(S)) * 1e-12;
      | K = Num_K / S;
  H : Inport
  P_pred : Inport  Port=2
  R : Inport  Port=3
  Add1 : Sum
  Cholesky Inverse : dspinverses/Cholesky Inverse  errmode=Warning
  H * P_pred * H' : Product  Inputs=3  Multiplication=Matrix(*)
  P_pred * H' : Product  Multiplication=Matrix(*)
  Transpose : Math  Operator=transpose
  avoid sing : Subsystem
  num_K / S : Product  Multiplication=Matrix(*)
  K : Outport
  wires:
  Transpose/1 -> H * P_pred * H'/3, P_pred * H'/2
  H/1 -> Transpose/1, H * P_pred * H'/1
  P_pred/1 -> H * P_pred * H'/2, P_pred * H'/1
  R/1 -> Add1/2
  H * P_pred * H'/1 -> Add1/1  "P_pred"
  Add1/1 -> avoid sing/1(S)  "S"
  Cholesky Inverse/1 -> num_K / S/2  "s^-1"
  P_pred * H'/1 -> num_K / S/1  "num_K"
  num_K / S/1 -> K/1
  avoid sing/1(S_) -> Cholesky Inverse/1

== system mainModel/MEKF ESTIMATION/MEASUREMENT/RESIDUALS ==
  note: if size(q_pred,1) > 1
      | q_pred = q_pred'; % metti in riga
      | end
      | dq = quatmultiply(quatconj(q_pred),q_meas);
      | if dq(1) < 0
      | dq = -dq; % evita ambiguita
      | end
  note: res_ss = dq(2:4) * 2;
      | b_pred = quatrotate(q_pred,b_meas_N);
      | res_mag = b_meas_B - b_pred;
      | b_pred_skew = [0 , -b_pred(3) , b_pred(2) ;
      | b_pred(3) , 0 , -b_pred(1) ;
      | -b_pred(2) , b_pred(1) , 0 ];
      |
      | y = [res_ss , res_mag]';
  q_meas : Inport
  q_pred : Inport  Port=2
  b_meas_B : Inport  Port=3
  b_real_N : Inport  Port=4
  Compare To Constant : simulink/Logic and Bit Operations/Compare To Constant  relop=>  const=0  OutDataTypeStr=boolean
  Gain : Gain  Gain=-1
  Gain1 : Gain  Gain=2
  Minus : Sum  Inputs=+-
  Quaternion Conjugate : aerolibutil/Quaternion Conjugate
  Quaternion Multiplication : aerolibutil/Quaternion Multiplication
  Quaternion Rotation : aerolibutil/Quaternion Rotation
  Reshape : Reshape  OutputDimensionality=Column vector (2-D)
  Reshape1 : Reshape  OutputDimensionality=Row vector (2-D)
  Reshape3 : Reshape  OutputDimensionality=Row vector (2-D)
  Reshape4 : Reshape  OutputDimensionality=Row vector (2-D)
  Selector : Selector  InputPortWidth=4  IndexOptions=Index vector (dialog)  Indices=1  OutputSizes=1
  Selector1 : Selector  InputPortWidth=4  IndexOptions=Index vector (dialog)  Indices=[2:4]  OutputSizes=1
  Switch : Switch  Criteria=u2 > Threshold  SaturateOnIntegerOverflow=off  InputSameDT=off
  Vector Concatenate : Concatenate  Mode=Multidimensional array  ConcatenateDimension=2
  y : Outport
  b_pred : Outport  Port=2
  wires:
  q_pred/1 -> Reshape1/1
  Reshape1/1 -> Quaternion Rotation/1, Quaternion Conjugate/1  "q_pred"
  Quaternion Conjugate/1 -> Quaternion Multiplication/1
  q_meas/1 -> Quaternion Multiplication/2
  Gain/1 -> Switch/3
  Quaternion Multiplication/1 -> Gain/1, Selector/1, Switch/1  "dq"
  Selector/1 -> Compare To Constant/1
  Compare To Constant/1 -> Switch/2
  Switch/1 -> Selector1/1  "dq"
  Selector1/1 -> Gain1/1
  Gain1/1 -> Vector Concatenate/1  "res_ss"
  Vector Concatenate/1 -> Reshape/1
  b_real_N/1 -> Reshape3/1
  Quaternion Rotation/1 -> b_pred/1, Minus/2  "b_pred_ B"
  b_meas_B/1 -> Reshape4/1
  Minus/1 -> Vector Concatenate/2
  Reshape3/1 -> Quaternion Rotation/2
  Reshape4/1 -> Minus/1  "b_meas_B"
  Reshape/1 -> y/1  "[res_ss ;  res_mag]"

== system mainModel/MEKF ESTIMATION/MEASUREMENT/SENSITIVITY MATRIX ==
  note: %% matrice di misura (H)
      | H_ss = [eye(3) , zeros(3)];
      | H_mag = [b_pred_skew , zeros(3,3)];
      | H = [H_ss ; H_mag];
  b_pred : Inport
  Constant : Constant  Value=eye(3)
  Constant1 : Constant  Value=zeros(3)
  Matrix Concatenate : Concatenate  Mode=Multidimensional array  ConcatenateDimension=2
  Matrix Concatenate1 : Concatenate  Mode=Multidimensional array  ConcatenateDimension=2
  Matrix Concatenate2 : Concatenate  Mode=Multidimensional array
  skewMatrix : Subsystem
  H : Outport
  wires:
  b_pred/1 -> skewMatrix/1(vect)  "b_pred"
  skewMatrix/1(skew) -> Matrix Concatenate/1  "b_pred_skew"
  Matrix Concatenate2/1 -> H/1
  Matrix Concatenate1/1 -> Matrix Concatenate2/1
  Matrix Concatenate/1 -> Matrix Concatenate2/2
  Constant/1 -> Matrix Concatenate1/1
  Constant1/1 -> Matrix Concatenate/2, Matrix Concatenate1/2

== system mainModel/MEKF ESTIMATION/PREDICTION/COVARIANCE MATRIX PROPAGATION ==
  note: P_pred = PHI * P_corr * PHI' + Q;
      | P_pred = 0.5 * (P_pred + P_pred');
  P_corr : Inport
  Add : Sum
  Add1 : Sum
  Constant1 : Constant  Value=MEKF.PHI
  Constant2 : Constant  Value=MEKF.Q
  Gain : Gain  Gain=1/2
  PHI * P_corr * PHI' : Product  Inputs=3  Multiplication=Matrix(*)
  Transpose : Math  Operator=transpose
  Transpose1 : Math  Operator=transpose
  P_pred : Outport
  wires:
  Transpose/1 -> PHI * P_corr * PHI'/3
  Add1/1 -> Add/1, Transpose1/1  "P_pred"
  Transpose1/1 -> Add/2
  Add/1 -> Gain/1
  Gain/1 -> P_pred/1
  PHI * P_corr * PHI'/1 -> Add1/1  "P_pred"
  Constant2/1 -> Add1/2
  Constant1/1 -> Transpose/1, PHI * P_corr * PHI'/1
  P_corr/1 -> PHI * P_corr * PHI'/2

== system mainModel/MEKF ESTIMATION/PREDICTION/STATE PROPAGATION ==
  note: % cinematica quaernione
      | w_corr_quat = [0, w_corr];
      | qDot_pred = 0.5 * quatmultiply(q_corr , w_corr_quat);
      | q_pred = q_corr + qDot_pred * dt;
      | q_pred = q_pred/norm(q_pred);
      | % dinamica sistema
      | wDot_pred = J \ (-cross(w_corr,J*w_corr') - cross(w_corr,h_RW) - hDot_RW + dist_Tq' + control_Tq)';
      | w_pred = w_corr + wDot_pred'*dt;
  q_corr : Inport
  w_corr : Inport  Port=2
  J : Inport  Port=3
  distTq : Inport  Port=4
  controlTq : Inport  Port=5
  hWheel : Inport  Port=6
  hDotWheel : Inport  Port=7
  QUATERNION KINEMATICS : Subsystem
  Reshape : Reshape  OutputDimensionality=Row vector (2-D)
  SYSTEM DYNAMICS : Subsystem
  q_pred : Outport
  w_pred : Outport  Port=2
  wires:
  J/1 -> SYSTEM DYNAMICS/2(J)
  hWheel/1 -> SYSTEM DYNAMICS/3(hWheel)
  hDotWheel/1 -> SYSTEM DYNAMICS/4(hDotWheel)
  distTq/1 -> SYSTEM DYNAMICS/5(distTq)
  controlTq/1 -> SYSTEM DYNAMICS/6(controlTq)
  SYSTEM DYNAMICS/1(w_pred) -> w_pred/1
  QUATERNION KINEMATICS/1(q_pred) -> q_pred/1
  w_corr/1 -> Reshape/1
  Reshape/1 -> SYSTEM DYNAMICS/1(w_corr), QUATERNION KINEMATICS/2(w_corr)
  q_corr/1 -> QUATERNION KINEMATICS/1(q_corr)

== system mainModel/TRIAD/attitudeDetermination_TRIAD/TRIAD - DCM determination ==
  note: Smatrix
  note: Vmatrix
  sMeas1 : Inport
  sMeas2 : Inport  Port=2
  r1 : Inport  Port=3
  r2 : Inport  Port=4
  Reshape{,1..3} (4 alike) : Reshape  OutputDimensionality=Column vector (2-D)
  Subsystem Reference : Subsystem  ReferencedSubsystem=vecNorm
  Subsystem Reference1 : Subsystem  ReferencedSubsystem=vecNorm
  Terminator : Terminator
  Terminator1 : Terminator
  Transpose : Math  Operator=transpose
  Vector Concatenate : Concatenate  NumInputs=3  Mode=Multidimensional array  ConcatenateDimension=2
  Vector Concatenate1 : Concatenate  NumInputs=3  Mode=Multidimensional array  ConcatenateDimension=2
  a x b : matrix_library/Cross Product
  a x v2 : matrix_library/Cross Product
  p x q : matrix_library/Cross Product
  p x s2 : matrix_library/Cross Product
  sMat *vMat : Product  Multiplication=Matrix(*)
  A_BN_est_TRIAD : Outport
  wires:
  sMat *vMat/1 -> A_BN_est_TRIAD/1
  r2/1 -> Reshape3/1  "b"
  sMeas1/1 -> Reshape/1  "p = s1"
  sMeas2/1 -> Reshape1/1  "q"
  p x q/1 -> Subsystem Reference/1
  Subsystem Reference/1 -> Terminator/1
  Subsystem Reference/2 -> Vector Concatenate1/2, p x s2/2  "s2"
  Subsystem Reference1/2 -> Vector Concatenate/2, a x v2/2  "v2"
  a x b/1 -> Subsystem Reference1/1
  Subsystem Reference1/1 -> Terminator1/1
  r1/1 -> Reshape2/1  "a = v1"
  a x v2/1 -> Vector Concatenate/3  "v3"
  p x s2/1 -> Vector Concatenate1/3  "s3"
  Vector Concatenate/1 -> Transpose/1  "vMat"
  Transpose/1 -> sMat *vMat/2  "vMat^t"
  Vector Concatenate1/1 -> sMat *vMat/1  "sMat"
  Reshape/1 -> Vector Concatenate1/1, p x s2/1, p x q/1
  Reshape3/1 -> a x b/2
  Reshape2/1 -> Vector Concatenate/1, a x v2/1, a x b/1
  Reshape1/1 -> p x q/2

== system mainModel/TRIAD/errorsTRIAD/angle error ==
  Aerr : Inport
  Acos : Trigonometry  Operator=acos
  Add : Sum  Inputs=+++
  Constant : Constant
  Constant1 : Constant
  Constant2 : Constant  Value=-1
  Gain : Gain  Gain=1/2
  Max : MinMax  Function=max  Inputs=2
  Min : MinMax  Inputs=2
  Minus1 : Sum  Inputs=+-
  Radians to Degrees : simulink_extras/Transformations/Radians to Degrees
  Scope : Scope
  Selector : Selector  NumberOfDimensions=2  InputPortWidth=3  IndexOptions=Index vector (dialog),Index vector (dialog)  Indices=1,1  OutputSizes=1,1
  Selector1 : Selector  NumberOfDimensions=2  InputPortWidth=3  IndexOptions=Index vector (dialog),Index vector (dialog)  Indices=2,2  OutputSizes=1,1
  Selector2 : Selector  NumberOfDimensions=2  InputPortWidth=3  IndexOptions=Index vector (dialog),Index vector (dialog)  Indices=3,3  OutputSizes=1,1
  theta_err : Outport
  wires:
  Aerr/1 -> Selector2/1, Selector/1, Selector1/1
  Selector1/1 -> Add/2
  Add/1 -> Minus1/1  "tr(Aerr)"
  Constant/1 -> Minus1/2
  Selector2/1 -> Add/3
  Minus1/1 -> Gain/1
  Selector/1 -> Add/1
  Acos/1 -> Scope/1, Radians to Degrees/1
  Radians to Degrees/1 -> theta_err/1
  Gain/1 -> Max/2
  Max/1 -> Min/1
  Min/1 -> Acos/1
  Constant2/1 -> Max/1
  Constant1/1 -> Min/2

== system mainModel/atmDrag/DRAG torque /Relative velocity body ==
  velRel_B : Inport
  om_B : Inport  Port=2
  rF : Inport  Port=3
  Reshape : Reshape  OutputDimensionality=Row vector (2-D)
  multipleCross : Subsystem
  vecSum : Subsystem
  vRelBody : Outport
  wires:
  om_B/1 -> Reshape/1
  rF/1 -> multipleCross/1(rF)
  Reshape/1 -> multipleCross/2(w_B)
  vecSum/1(prod) -> vRelBody/1
  multipleCross/1(vRelFaces) -> vecSum/2(vRelFaces)
  velRel_B/1 -> vecSum/1(vRel_B)

== system mainModel/atmDrag/DRAG torque /dragForce ==
  rho : Inport
  vRelBody : Inport  Port=2
  Nb : Inport  Port=3
  A : Inport  Port=4
  Gain : Gain  Gain=-1/2
  Gain1 : Gain  Gain=pert.drag.CD
  Gain2 : Gain  Gain=1e3
  Product : Product  Inputs=4
  Reshape : Reshape
  Square : Math  Operator=square
  Sum of Elements : Sum  Inputs=+  CollapseMode=Specified dimension
  To Workspace : ToWorkspace  VariableName=dragForce  SampleTime=-1
  multipleDotProd : Subsystem
  multipleVecNorm : Subsystem
  multipleVecNorm3 : Subsystem  Commented=on
  multipleVersVec : Subsystem
  vecProd : Subsystem
  F : Outport
  wires:
  rho/1 -> Gain/1
  Gain/1 -> Gain1/1
  Nb/1 -> multipleDotProd/1(Nbvect)
  Gain2/1 -> Square/1
  multipleVecNorm/1(normVec) -> multipleVersVec/2(normVec), Gain2/1
  Square/1 -> Product/2
  multipleVersVec/1(versVec) -> vecProd/2(versVec), multipleDotProd/2(vers)
  multipleDotProd/1(visionVec) -> Product/3
  Product/1 -> vecProd/1(constVec)
  vecProd/1(Fvect) -> Sum of Elements/1, F/1
  vRelBody/1 -> multipleVersVec/1(vRelBody), multipleVecNorm/1(vRelBody)
  Gain1/1 -> Product/1
  A/1 -> Product/4
  Sum of Elements/1 -> Reshape/1
  Reshape/1 -> To Workspace/1

== system mainModel/atmDrag/DRAG torque /dragTorque ==
  Fvect : Inport
  rFvect : Inport  Port=2
  Minus : Sum  Inputs=-+
  Minus1 : Sum  Inputs=-+
  Minus2 : Sum  Inputs=+-
  Product{,1..5} (6 alike) : Product
  Selector : Selector  NumberOfDimensions=2  InputPortWidth=3  IndexOptions=Select all,Index vector (dialog)  Indices=[1 3],1  OutputSizes=1,1
  Selector1 : Selector  NumberOfDimensions=2  InputPortWidth=3  IndexOptions=Select all,Index vector (dialog)  Indices=[1 3],2  OutputSizes=1,1
  Selector2 : Selector  NumberOfDimensions=2  InputPortWidth=3  IndexOptions=Select all,Index vector (dialog)  Indices=[1 3],3  OutputSizes=1,1
  Selector3 : Selector  NumberOfDimensions=2  InputPortWidth=3  IndexOptions=Select all,Index vector (dialog)  Indices=[1 3],1  OutputSizes=1,1
  Selector4 : Selector  NumberOfDimensions=2  InputPortWidth=3  IndexOptions=Select all,Index vector (dialog)  Indices=[1 3],2  OutputSizes=1,1
  Selector5 : Selector  NumberOfDimensions=2  InputPortWidth=3  IndexOptions=Select all,Index vector (dialog)  Indices=[1 3],3  OutputSizes=1,1
  Sum of Elements : Sum  Inputs=+  CollapseMode=Specified dimension
  Vector Concatenate : Concatenate  NumInputs=3  Mode=Multidimensional array  ConcatenateDimension=2
  DRAG : Outport
  dragMATRIX : Outport  Port=2
  wires:
  rFvect/1 -> Selector2/1, Selector1/1, Selector/1
  Fvect/1 -> Selector5/1, Selector4/1, Selector3/1
  Selector/1 -> Product2/1, Product/1  "rfx"
  Selector1/1 -> Product5/1, Product1/2  "rfy"
  Selector2/1 -> Product4/1, Product3/1  "rfz"
  Selector3/1 -> Product1/1, Product3/2  "fx"
  Selector4/1 -> Product/2, Product4/2  "fy"
  Selector5/1 -> Product5/2, Product2/2  "fz"
  Product4/1 -> Minus/1  "rfz*fy"
  Product5/1 -> Minus/2  "rfy*fz"
  Product3/1 -> Minus1/2  "rfz*fx"
  Product2/1 -> Minus1/1  "rfx*fz"
  Product/1 -> Minus2/1  "rfx*fy"
  Product1/1 -> Minus2/2  "rfy*fx"
  Vector Concatenate/1 -> dragMATRIX/1, Sum of Elements/1
  Minus1/1 -> Vector Concatenate/2
  Minus2/1 -> Vector Concatenate/3
  Minus/1 -> Vector Concatenate/1
  Sum of Elements/1 -> DRAG/1

== system mainModel/atmDrag/DRAG torque /vecCrossOld ==
  rFvect : Inport
  Fvect : Inport  Port=2
  Cross Product{,1..9} (10 alike) : matrix_library/Cross Product
  Subsystem : Subsystem
  Subsystem1 : Subsystem
  Sum of Elements : Sum  Inputs=+  CollapseMode=Specified dimension
  Vector Concatenate : Concatenate  NumInputs=10  Mode=Multidimensional array
  DRAG : Outport
  DRAGmatrix : Outport  Port=2
  wires:
  Cross Product2/1 -> Vector Concatenate/3
  Cross Product5/1 -> Vector Concatenate/5
  Cross Product1/1 -> Vector Concatenate/2
  Cross Product/1 -> Vector Concatenate/1
  Cross Product7/1 -> Vector Concatenate/8
  Cross Product8/1 -> Vector Concatenate/9
  Cross Product3/1 -> Vector Concatenate/4
  Cross Product4/1 -> Vector Concatenate/6
  Cross Product6/1 -> Vector Concatenate/7
  Cross Product9/1 -> Vector Concatenate/10
  rFvect/1 -> Subsystem/1(Fvect)  "Fvect"
  Subsystem/1(F1) -> Cross Product/1
  Subsystem/2(F2) -> Cross Product1/1
  Subsystem/3(F3) -> Cross Product2/1
  Subsystem/4(F4) -> Cross Product3/1
  Subsystem/5(F5) -> Cross Product5/1
  Subsystem/6(F6) -> Cross Product4/1
  Subsystem/7(F7) -> Cross Product6/1
  Subsystem/8(F8) -> Cross Product7/1
  Subsystem/9(F9) -> Cross Product8/1
  Subsystem/10(F10) -> Cross Product9/1
  Fvect/1 -> Subsystem1/1(In1)
  Subsystem1/10(rF10) -> Cross Product9/2
  Subsystem1/9(rF9) -> Cross Product8/2
  Subsystem1/8(rF8) -> Cross Product7/2
  Subsystem1/7(rF7) -> Cross Product6/2
  Subsystem1/6(rF6) -> Cross Product4/2
  Subsystem1/5(rF5) -> Cross Product5/2
  Subsystem1/4(rF4) -> Cross Product3/2
  Subsystem1/3(rF3) -> Cross Product2/2
  Subsystem1/2(rF2) -> Cross Product1/2
  Subsystem1/1(rF1) -> Cross Product/2
  Vector Concatenate/1 -> DRAGmatrix/1, Sum of Elements/1
  Sum of Elements/1 -> DRAG/1
